simulink model "PBCforHESSsemiactive"  (R2023a)
settings: Solver=ode4  StartTime=0.0  StopTime=10.0  FixedStep=1/350000  RelTol=1e-3
undefined symbols (not defined in the file): Acid, Lead
libraries: spsFirstOrderFilterLib x5, spsSeriesRLCBranchLib x5, spsCurrentMeasurementLib x4, spsGroundLib x3, spsControlledCurrentSourceLib x2, spsIGBTDiodeLib x2, spsPWMGeneratorDCDCLib x2, spsVoltageMeasurementLib x2, spsBatteryLib x1, spsControlledVoltageSourceLib x1, spsIdealSwitchLib x1, spsSupercapacitorLib x1
settings Model: Creator=USUARIO  LastModifiedBy=USUARIO

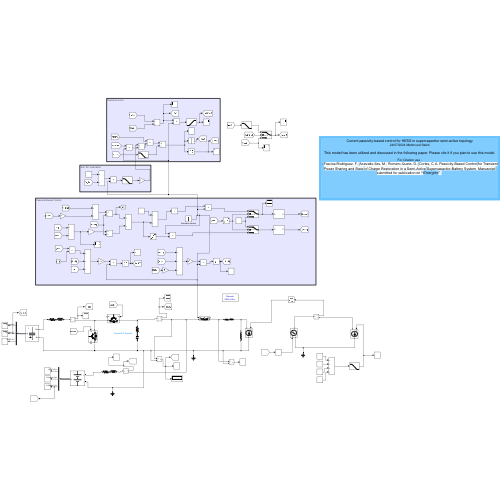
[thumbnail: Simulink's stored preview of the top-level diagram]
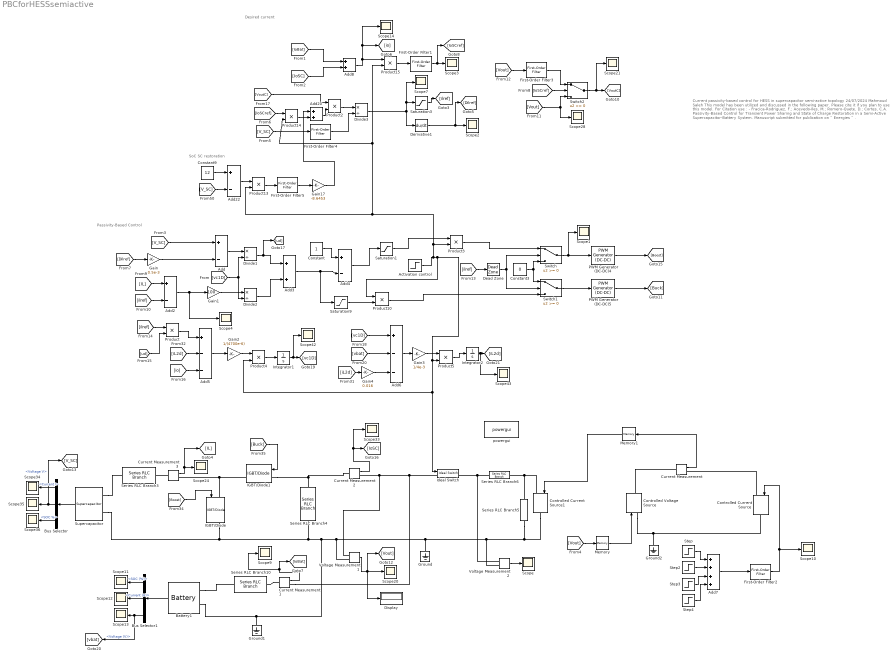
== system PBCforHESSsemiactive ==
  note: Passivity-Based Control
  note: SoC SC restoration
  note: Desired current
  note: Current passivity-based control for HESS in supercapacitor semi-active topology
      | 24/07/2024 Mahmoud Saleh
      |
      | This model has been utilized and discussed in the following paper. Please cite it if you plan to use this model.
      |
      | For Citation use :
      | - Fracica-Rodriguez, F.; Acevedo-Iles, M.; Romero-Quete, D.; Cortes, C.A. Passivity-Based Control for Transient Power Sharing and State of Charge Restoration in a Semi-Active Supercapacitor-Battery System. Manuscript submitted for publication on “ Energies ” .
  Activation control : Step  Time=3  SampleTime=0
  Add{,2,4,22} (4 alike) : Sum  Inputs=+-
  Add20 : Sum
  Add3 : Sum
  Add5 : Sum  Inputs=+--
  Add6 : Sum  Inputs=+--
  Add7 : Sum  Inputs=++++
  Add8 : Sum
  Battery1 : spsBatteryLib/Battery  BatType=Lead-Acid  ShowTempParam=off  ThermalPreset=no  ShowAgeParam=off  NomV=24  NomQ=100  SOC=40  Batt_Tr=30  PresetModel=on  MaxQ=104.1667  MinV=18  FullV=26.1316  Dis_rate=20  R=0.0024  Normal_OP=31.0278  expZone="[24.4342     0.333333]"  current=[6.5 13 32.5]  Units=Time  Tci=20  NomT=20  T2=-30  MaxQ2=4.8  FullV2=7.1  Normal_OP2=5.655  expZone2="[6.58           1]"  Rca=0.6  ti=2000  Dp=0  Neq0=0  Tsim=1e6  Ta1=25  Qeol=5.4*0.9  Reol=0.013333*1.2  Char_age=[2.3478, 3]  Dis_age=[2.3478, 10]  N1=1500  N2=10500  N3=1000  N4=1400  Ta2=45  N5=950
  Bus Selector : BusSelector  OutputSignals=Current I,Voltage V,SOC %
  Bus Selector1 : BusSelector  OutputSignals=SOC (%),Current (A),Voltage (V)
  Constant : Constant
  Constant3 : Constant  Value=0
  Constant9 : Constant  Value=12
  Controlled Current Source : spsControlledCurrentSourceLib/Controlled Current Source  Initialize=off  Source_Type=DC  Amplitude=1  Phase=0  Frequency=0  Measurements=None
  Controlled Current Source1 : spsControlledCurrentSourceLib/Controlled Current Source  Initialize=off  Source_Type=DC  Amplitude=1  Phase=0  Frequency=0  Measurements=None
  Controlled Voltage Source : spsControlledVoltageSourceLib/Controlled Voltage Source  Initialize=off  Source_Type=DC  Amplitude=0  Phase=0  Frequency=0  Measurements=None
  Current Measurement{,1..3} (4 alike) : spsCurrentMeasurementLib/Current Measurement  PhasorSimulation=off  OutputType=Complex  PSBequivalent=0
  Dead Zone : DeadZone  LowerValue=-0.05  UpperValue=0.05
  Derivative1 : Derivative
  Display : Display
  Divide1 : Product  Inputs=*/
  Divide2 : Product  Inputs=*/
  Divide3 : Product  Inputs=*/
  First-Order Filter1 : spsFirstOrderFilterLib/First-Order Filter  FilterType=Highpass  Tc=20e-2*5  Ts=0  Initialize=off  Vac_Init=[0, 0, 60]  Vdc_Init=0  PlotResponse=off  FreqRange="[0,  200,  1]"
  First-Order Filter2 : spsFirstOrderFilterLib/First-Order Filter  FilterType=Lowpass  Tc=0.001/5  Ts=0  Initialize=on  Vac_Init=[0, 0, 60]  Vdc_Init=0  PlotResponse=off  FreqRange="[0,  200,  1]"
  First-Order Filter3 : spsFirstOrderFilterLib/First-Order Filter  FilterType=Lowpass  Tc=10e-4  Ts=0  Initialize=on  Vac_Init=[0, 0, 60]  Vdc_Init=23.57  PlotResponse=off  FreqRange="[0,  200,  1]"
  First-Order Filter4 : spsFirstOrderFilterLib/First-Order Filter  FilterType=Lowpass  Tc=10e-4  Ts=0  Initialize=on  Vac_Init=[0, 0, 60]  Vdc_Init=12  PlotResponse=off  FreqRange="[0,  200,  1]"
  First-Order Filter5 : spsFirstOrderFilterLib/First-Order Filter  FilterType=Lowpass  Tc=1.2  Ts=0  Initialize=on  Vac_Init=[0, 0, 60]  Vdc_Init=0  PlotResponse=off  FreqRange="[0,  200,  1]"
  Gain : Gain  Gain=0.5e-3
  Gain1 : Gain  Gain=100
  Gain17 : Gain  Gain=-8.6453
  Gain2 : Gain  Gain=1/(4700e-6)
  Gain3 : Gain  Gain=1/4e-3
  Gain4 : Gain  Gain=0.016
  Ground : spsGroundLib/Ground  LConnTagsString=a
  Ground1 : spsGroundLib/Ground  LConnTagsString=a
  Ground2 : spsGroundLib/Ground  LConnTagsString=a
  IGBT/Diode : spsIGBTDiodeLib/IGBT//Diode  Ron=1e-3  Rs=1e5  Cs=inf  Measurements=on
  IGBT/Diode1 : spsIGBTDiodeLib/IGBT//Diode  Ron=1e-3  Rs=1e5  Cs=inf  Measurements=on
  Ideal Switch : spsIdealSwitchLib/Ideal Switch  Ron=0.001  Lon=0  IC=0  Rs=1e6  Cs=inf  Measurements=on
  Integrator1 : Integrator  InitialCondition=23.57  LimitOutput=on  UpperSaturationLimit=26  LowerSaturationLimit=19
  Integrator2 : Integrator  InitialCondition=0.5  LimitOutput=on  UpperSaturationLimit=30  LowerSaturationLimit=-30
  Memory : Memory
  Memory1 : Memory
  PWM Generator (DC-DC)4 : spsPWMGeneratorDCDCLib/PWM Generator (DC-DC)  Fsw=35000  Ts=0
  PWM Generator (DC-DC)5 : spsPWMGeneratorDCDCLib/PWM Generator (DC-DC)  Fsw=35000  Ts=0
  Product{,2..5,10,13..15} (9 alike) : Product
  Saturation1 : Saturate  UpperLimit=1  LowerLimit=0
  Saturation3 : Saturate  UpperLimit=50  LowerLimit=-50
  Saturation9 : Saturate  UpperLimit=1  LowerLimit=0
  Scope{,1..4,7,9..14,20..21,24,28,33..36,42..43} (22 alike) : Scope
  Series RLC Branch10 : spsSeriesRLCBranchLib/Series RLC Branch  LConnTagsString=__new0  RConnTagsString=__new0  BranchType=RL  Resistance=1e-3  Inductance=6e-3  SetiL0=off  InitialCurrent=0  Capacitance=1e-6  Setx0=off  InitialVoltage=0  Measurements=None
  Series RLC Branch3 : spsSeriesRLCBranchLib/Series RLC Branch  LConnTagsString=__new0  RConnTagsString=__new0  BranchType=RL  Resistance=1e-3  Inductance=0.5e-3  SetiL0=off  InitialCurrent=0  Capacitance=1e-6  Setx0=off  InitialVoltage=0  Measurements=None
  Series RLC Branch4 : spsSeriesRLCBranchLib/Series RLC Branch  LConnTagsString=__new0  RConnTagsString=__new0  BranchType=RC  Resistance=1e-3  Inductance=1e-3  SetiL0=off  InitialCurrent=0  Capacitance=4700e-6  Setx0=on  InitialVoltage=23.57  Measurements=None
  Series RLC Branch5 : spsSeriesRLCBranchLib/Series RLC Branch  LConnTagsString=__new0  RConnTagsString=__new0  BranchType=R  Resistance=1e4  Inductance=1e-3  SetiL0=off  InitialCurrent=0  Capacitance=4700e-6  Setx0=off  InitialVoltage=0  Measurements=None
  Series RLC Branch6 : spsSeriesRLCBranchLib/Series RLC Branch  LConnTagsString=__new0  RConnTagsString=__new0  BranchType=RL  Resistance=1e-4  Inductance=75e-6  SetiL0=off  InitialCurrent=0  Capacitance=4700e-6  Setx0=off  InitialVoltage=0  Measurements=None
  Step : Step  Time=10  Before=1  After=15  SampleTime=0
  Step2 : Step  Time=30  After=-10  SampleTime=0
  Step3 : Step  Time=50  After=-20  SampleTime=0
  Step4 : Step  Time=70  After=15  SampleTime=0
  Supercapacitor : spsSupercapacitorLib/Supercapacitor  C=83  Rdc=6e-3  Voltage=16  Ns=6  Np=1  Vinit=12  Temp=25  PresetModel=off  EstParam=off  Nc=1  r=1e-9  epsilon=6.0208e-10  Ich=10  Vstern="[0.161  2.7  7.8]"  Self_dis=on  Ioc=10  Vself="[48  47.8  47.06  44.65]"  demandeplot=off  I="[10  20 100  500]"  Units=sec  Vmax=0  If=0  deltaV=0  alpha=0  sec=0
      settings: LibrarySourceBlock=sps_lib/Sources/Supercapacitor
  Switch : Switch  SaturateOnIntegerOverflow=off  InputSameDT=off
  Switch1 : Switch  SaturateOnIntegerOverflow=off  InputSameDT=off
  Switch2 : Switch  SaturateOnIntegerOverflow=off  InputSameDT=off
  Voltage Measurement1 : spsVoltageMeasurementLib/Voltage Measurement  PhasorSimulation=off  OutputType=Complex  PSBequivalent=0
  Voltage Measurement2 : spsVoltageMeasurementLib/Voltage Measurement  PhasorSimulation=off  OutputType=Complex  PSBequivalent=0
  powergui : spspowerguiLib/powergui  Priority=1  SimulationMode=Discrete  SampleTime=1/350000  frequency=60  Iterations=50  frequencyindice=0  Pbase=100e6  ErrMax=1e-4  UnitsV=kV  UnitsW=MW  buscounter=0  FunctionMessages=off  echomessages=off  EnableUseOfTLC=off  CurrentSourceSwitches=off  DisableSnubberDevices=off  DisableRonSwitches=off  DisableVfSwitches=off  DisplayEquations=off  AutomaticDiscreteSolvers=off  SolverType=Tustin/Backward Euler (TBE)  Interpol=off  ExternalGateDelay=off  methode=off  Ts=100  x0status=blocks  SPID=on  SwTol=0  HookPort=off  NonlinearTolerance=1e-4  nMaxIteration=100  ContinueOnMaxIteration=off  RestoreLinks=warning  ResistiveCurrentMeasurement=off  Frange=[0:2:500]  Ylog=off  Xlog=on  ShowGrid=off  save=off  variable=ZData  structure=0  ZoomFFT=off  StartTime=0.0  cycles=1  DisplayStyle=1  fundamental=60  FreqAxis=off  MaxFrequency=1000  frequencyindicesteady=1  RmsSteady=1  display=off
  wires:
  First-Order Filter3/1 -> Switch2/1
  Bus Selector/2 -> [V_SC], Scope35/1  "<Voltage V>"
  First-Order Filter4/1 -> Divide3/2
  Integrator2/1 -> Scope43/1, [iL2d]
  Gain17/1 -> Add20/1
  [Vout] -> Scope28/1, Switch2/3
  Switch2/1 -> Scope21/1, [VoutC]
  PWM Generator (DC-DC)5/1 -> [Buck]
  Divide1/1 -> [ud], Add3/1
  [IoSCref] -> Product14/1
  Add7/1 -> First-Order Filter2/1
  Gain2/1 -> Product4/1
  [Buck] -> IGBT/Diode1/1
  Add22/1 -> Product13/1
  Saturation9/1 -> Product10/2
  [Vout] -> First-Order Filter3/1
  [IL] -> Add2/1
  Saturation1/1 -> Product3/1
  Current Measurement/1 -> Memory1/1
  Product14/1 -> Add20/2
  Step3/1 -> Add7/3
  Gain3/1 -> Product5/1
  Voltage Measurement2/1 -> Scope/1
  Voltage Measurement1/1 -> [Vout], Display/1, Scope20/1
  [iL2d] -> Gain4/1
  Product13/1 -> First-Order Filter5/1
  [VoutC] -> Product2/1
  [IoSCref] -> Switch2/2
  Switch/1 -> Scope1/1, PWM Generator (DC-DC)4/1
  Add20/1 -> Product2/2
  [ilref] -> Dead Zone/1
  [io] -> Add5/3
  Divide3/1 -> Derivative1/1, Scope7/1, Saturation3/1
  [V_SC] -> Add22/2
  Product15/1 -> First-Order Filter1/1
  Product10/1 -> Switch1/3
  Product3/1 -> Switch/1
  Dead Zone/1 -> Switch1/2, Switch/2
  PWM Generator (DC-DC)4/1 -> [Boost]
  Derivative1/1 -> [Dilref], Scope2/1
  [IoSC] -> Add8/2
  Product4/1 -> Integrator1/1
  Activation control/1 -> Product13/2, Product14/2, Product15/2, Product3/2, Ideal Switch/1, Product4/2, Product5/2, Product10/1
  Product5/1 -> Integrator2/1
  Constant/1 -> Add4/1
  [ilref] -> Product/1
  Switch1/1 -> PWM Generator (DC-DC)5/1
  [vbat] -> Add6/2
  Gain/1 -> Add/2
  [V_SC] -> First-Order Filter4/1
  [ud] -> Product/2
  Product/1 -> Add5/1
  Memory1/1 -> Controlled Current Source1/1
  Integrator1/1 -> Scope42/1, [vc1D]
  Constant3/1 -> Switch1/1, Switch/3
  [Vout] -> Memory/1
  [iL2d] -> Add5/2
  [vc1D] -> Divide2/2, Divide1/2
  Saturation3/1 -> [ilref]
  Add2/1 -> Scope4/1, Gain1/1
  Divide2/1 -> Add3/2
  Gain1/1 -> Divide2/1
  Step4/1 -> Add7/4
  Constant9/1 -> Add22/1
  First-Order Filter1/1 -> [IoSCref], Scope3/1
  Product2/1 -> Divide3/1
  Add3/1 -> Saturation9/1, Add4/2
  [Dilref] -> Gain/1
  Add/1 -> Divide1/1
  Battery1/1 -> Bus Selector1/1
  Bus Selector/3 -> Scope36/1  "<SOC %>"
  Current Measurement2/1 -> [IoSC], Scope33/1
  [V_SC] -> Add/1
  [ilref] -> Add2/2
  Bus Selector1/3 -> [vbat], Scope13/1  "<Voltage (V)>"
  Bus Selector/1 -> Scope34/1  "<Current I>"
  Bus Selector1/1 -> Scope11/1  "<SOC (%)>"
  [vc1D] -> Add6/1
  Memory/1 -> Controlled Voltage Source/1
  Supercapacitor/1 -> Bus Selector/1
  Bus Selector1/2 -> Scope12/1  "<Current (A)>"
  [Boost] -> IGBT/Diode/1
  Add8/1 -> Product15/1, Scope14/1, [io]
  First-Order Filter2/1 -> Scope10/1, Controlled Current Source/1
  Current Measurement3/1 -> [IL], Scope24/1
  Add5/1 -> Gain2/1
  [IoBat] -> Add8/1
  Current Measurement1/1 -> Scope9/1, [IoBat]
  Step2/1 -> Add7/2
  Add6/1 -> Gain3/1
  Step/1 -> Add7/1
  Gain4/1 -> Add6/3
  Add4/1 -> Saturation1/1
  First-Order Filter5/1 -> Gain17/1
  connections:
  Current Measurement2/RConn1 -- Current Measurement1/RConn1 -- Ideal Switch/LConn1 -- Voltage Measurement1/LConn1
  Series RLC Branch5/RConn1 -- Controlled Current Source1/RConn1 -- Series RLC Branch4/RConn1 -- Supercapacitor/LConn2 -- IGBT/Diode/RConn1 -- Battery1/LConn2 -- Ground1/LConn1 -- Voltage Measurement1/LConn2 -- Ground/LConn1 -- Voltage Measurement2/LConn2
  IGBT/Diode1/LConn1 -- Series RLC Branch4/LConn1 -- Current Measurement2/LConn1
  Ideal Switch/RConn1 -- Series RLC Branch6/LConn1 -- Voltage Measurement2/LConn1
  Series RLC Branch5/LConn1 -- Series RLC Branch6/RConn1 -- Controlled Current Source1/LConn1
  Controlled Voltage Source/LConn1 -- Controlled Current Source/RConn1 -- Ground2/LConn1
  Current Measurement3/RConn1 -- IGBT/Diode/LConn1 -- IGBT/Diode1/RConn1
  Controlled Current Source/LConn1 -- Current Measurement/RConn1
  Supercapacitor/LConn1 -- Series RLC Branch3/LConn1
  Battery1/LConn1 -- Series RLC Branch10/LConn1
  Current Measurement3/LConn1 -- Series RLC Branch3/RConn1
  Current Measurement1/LConn1 -- Series RLC Branch10/RConn1
  Controlled Voltage Source/RConn1 -- Current Measurement/LConn1
